simulink library "BMSI_lib"  (Simulink 7.5)
settings: Solver=ode45  StartTime=0.0  StopTime=10.0  RelTol=1e-3
values from neighbouring files (symbols this model uses):
  pBMSI_bool_HandShakeOverFlag_C = Simulink.Parameter    [BMSI_par.m]
  pBMSI_bool_InterLockOverFlag_C = Simulink.Parameter    [BMSI_par.m]
  pBMSI_bool_StnCfgStOverFlag_C = Simulink.Parameter    [BMSI_par.m]
  pBMSI_mV_DSPInterLowrRngThd_C = Simulink.Parameter    [BMSI_par.m]
  pBMSI_mV_DSPInterUpprRngThd_C = Simulink.Parameter    [BMSI_par.m]
  pBMSI_mV_InterlockDiffThd_C = Simulink.Parameter    [BMSI_par.m]
  pBMSI_mV_InterlockLowrRngThd_C = Simulink.Parameter    [BMSI_par.m]
  pBMSI_mV_InterlockUpprRngThd_C = Simulink.Parameter    [BMSI_par.m]
  pBMSI_pct_LoSOCThd_C = Simulink.Parameter    [BMSI_par.m]
  pBMSI_st_DCChrgrErrSt_C = Simulink.Parameter    [BMSI_par.m]
undefined symbols (not defined in the file or in its folder): ChrgHandShakeTyp, ChrgStationParCnfTyp, FAWBatInsMeasStsTyp, FAWBmsChrgStsTyp, FAWBmsContErrTyp, FAWBMSStsTyp, p_bool_dSPaceEnbl_C, p_bool_False_M, p_bool_True_M
libraries: BaseOperationLib_Browser x116, PES_CZ_FAW x15, simulink x1
(part 1 of 2)
settings Model: Creator=wuaibin  LastModifiedBy=wuaibin

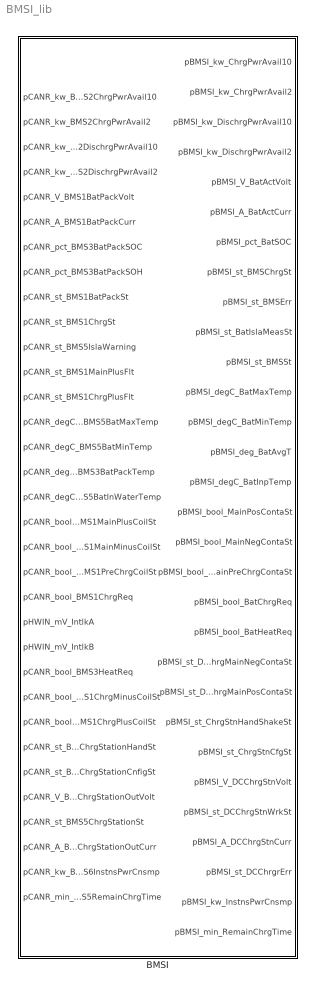
== system BMSI_lib ==
  BMSI : Subsystem  TreatAsAtomicUnit=on

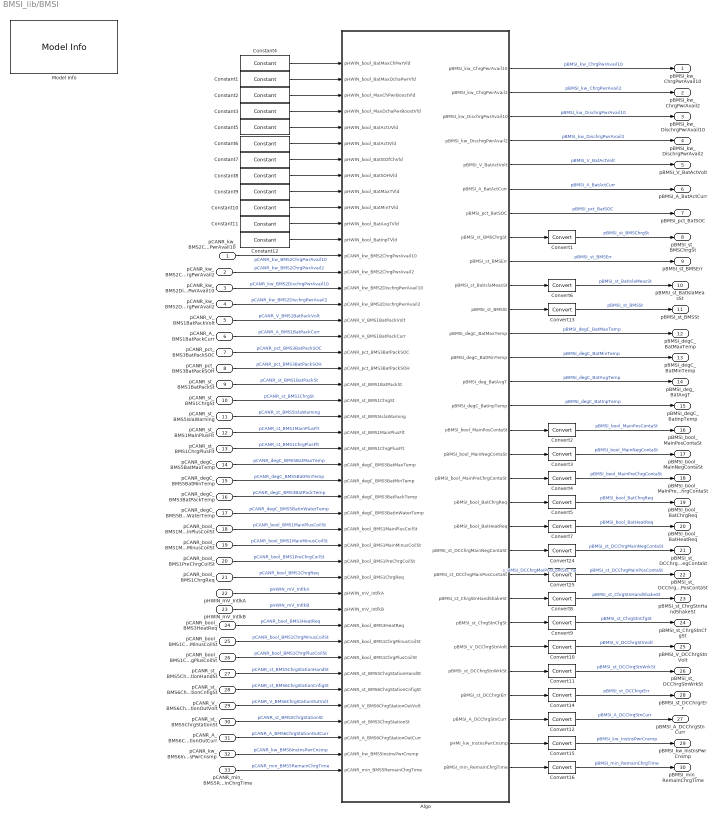
== system BMSI_lib/BMSI ==
  pCANR_kw_BMS2ChrgPwrAvail10 : Inport  OutDataType=fixdt(1, 16)  OutScaling=2^0
  pCANR_kw_BMS2ChrgPwrAvail2 : Inport  Port=2  OutDataType=fixdt(1, 16)  OutScaling=2^0
  pCANR_kw_BMS2DischrgPwrAvail10 : Inport  Port=3  OutDataType=fixdt(1, 16)  OutScaling=2^0
  pCANR_kw_BMS2DischrgPwrAvail2 : Inport  Port=4  OutDataType=fixdt(1, 16)  OutScaling=2^0
  pCANR_V_BMS1BatPackVolt : Inport  Port=5  OutDataType=fixdt(1, 16)  OutScaling=2^0
  pCANR_A_BMS1BatPackCurr : Inport  Port=6  OutDataType=fixdt(1, 16)  OutScaling=2^0
  pCANR_pct_BMS3BatPackSOC : Inport  Port=7  OutDataType=fixdt(1, 16)  OutScaling=2^0
  pCANR_pct_BMS3BatPackSOH : Inport  Port=8  OutDataType=fixdt(1, 16)  OutScaling=2^0
  pCANR_st_BMS1BatPackSt : Inport  Port=9  OutDataType=fixdt(1, 16)  OutScaling=2^0
  pCANR_st_BMS1ChrgSt : Inport  Port=10  OutDataType=fixdt(1, 16)  OutScaling=2^0
  pCANR_st_BMS5IslaWarning : Inport  Port=11  OutDataType=fixdt(1, 16)  OutScaling=2^0
  pCANR_st_BMS1MainPlusFlt : Inport  Port=12  OutDataType=fixdt(1, 16)  OutScaling=2^0
  pCANR_st_BMS1ChrgPlusFlt : Inport  Port=13  OutDataType=fixdt(1, 16)  OutScaling=2^0
  pCANR_degC_BMS5BatMaxTemp : Inport  Port=14  OutDataType=fixdt(1, 16)  OutScaling=2^0
  pCANR_degC_BMS5BatMinTemp : Inport  Port=15  OutDataType=fixdt(1, 16)  OutScaling=2^0
  pCANR_degC_BMS3BatPackTemp : Inport  Port=16  OutDataType=fixdt(1, 16)  OutScaling=2^0
  pCANR_degC_BMS5BatInWaterTemp : Inport  Port=17  OutDataType=fixdt(1, 16)  OutScaling=2^0
  pCANR_bool_BMS1MainPlusCoilSt : Inport  Port=18  OutDataType=fixdt(1, 16)  OutScaling=2^0
  pCANR_bool_BMS1MainMinusCoilSt : Inport  Port=19  OutDataType=fixdt(1, 16)  OutScaling=2^0
  pCANR_bool_BMS1PreChrgCoilSt : Inport  Port=20  OutDataType=fixdt(1, 16)  OutScaling=2^0
  pCANR_bool_BMS1ChrgReq : Inport  Port=21  OutDataType=fixdt(1, 16)  OutScaling=2^0
  pHWIN_mV_IntlkA : Inport  Port=22  OutDataType=fixdt(1, 16)  OutScaling=2^0
  pHWIN_mV_IntlkB : Inport  Port=23  OutDataType=fixdt(1, 16)  OutScaling=2^0
  pCANR_bool_BMS3HeatReq : Inport  Port=24  OutDataType=fixdt(1, 16)  OutScaling=2^0
  pCANR_bool_BMS1ChrgMinusCoilSt : Inport  Port=25  OutDataType=fixdt(1, 16)  OutScaling=2^0
  pCANR_bool_BMS1ChrgPlusCoilSt : Inport  Port=26  OutDataType=fixdt(1, 16)  OutScaling=2^0
  pCANR_st_BMS5ChrgStationHandSt : Inport  Port=27  OutDataType=fixdt(1, 16)  OutScaling=2^0
  pCANR_st_BMS6ChrgStationCnfigSt : Inport  Port=28  OutDataType=fixdt(1, 16)  OutScaling=2^0
  pCANR_V_BMS6ChrgStationOutVolt : Inport  Port=29  OutDataType=fixdt(1, 16)  OutScaling=2^0
  pCANR_st_BMS5ChrgStationSt : Inport  Port=30  OutDataType=fixdt(1, 16)  OutScaling=2^0
  pCANR_A_BMS6ChrgStationOutCurr : Inport  Port=31  OutDataType=fixdt(1, 16)  OutScaling=2^0
  pCANR_kw_BMS6InstnsPwrCnsmp : Inport  Port=32  OutDataType=fixdt(1, 16)  OutScaling=2^0
  pCANR_min_BMS5RemainChrgTime : Inport  Port=33  OutDataType=fixdt(1, 16)  OutScaling=2^0
  Algo : Subsystem
  Constant{1..12} (12 alike) : BaseOperationLib_Browser/Sources&Sinks/Constant  Value=p_bool_True_M  OutMin=[]  OutMax=[]  OutDataTypeMode=uint32  OutDataType=fixdt(1, 16)  ConRadixGroup=Use specified scaling  OutScaling=2^0  OutDataTypeStr=uint32
  Convert{1..16,24..25} (18 alike) : DataTypeConversion  OutDataType=fixdt(1, 16)  OutScaling=2^0
  Model Info : simulink/Model-Wide Utilities/Model Info  SystemSampleTime=-1  InitialBlockCM=None  BlockCM=None  Frame=on  DisplayStringWithTags=Model Info\nCreated: %<Created>\nCreator: %<Creator>  HorizontalTextAlignment=Center  LeftAlignmentValue=0.5  SourceBlockDiagram=HQEV_HCU  TagMaxNumber=20
  pBMSI_kw_ChrgPwrAvail10 : Outport  OutDataType=fixdt(1, 16)  OutScaling=2^0
  pBMSI_kw_ChrgPwrAvail2 : Outport  Port=2  OutDataType=fixdt(1, 16)  OutScaling=2^0
  pBMSI_kw_DischrgPwrAvail10 : Outport  Port=3  OutDataType=fixdt(1, 16)  OutScaling=2^0
  pBMSI_kw_DischrgPwrAvail2 : Outport  Port=4  OutDataType=fixdt(1, 16)  OutScaling=2^0
  pBMSI_V_BatActVolt : Outport  Port=5  OutDataType=fixdt(1, 16)  OutScaling=2^0
  pBMSI_A_BatActCurr : Outport  Port=6  OutDataType=fixdt(1, 16)  OutScaling=2^0
  pBMSI_pct_BatSOC : Outport  Port=7  OutDataType=fixdt(1, 16)  OutScaling=2^0
  pBMSI_st_BMSChrgSt : Outport  Port=8  OutDataType=fixdt(1, 16)  OutScaling=2^0
  pBMSI_st_BMSErr : Outport  Port=9  OutDataType=fixdt(1, 16)  OutScaling=2^0
  pBMSI_st_BatIslaMeasSt : Outport  Port=10  OutDataType=fixdt(1, 16)  OutScaling=2^0
  pBMSI_st_BMSSt : Outport  Port=11  OutDataType=fixdt(1, 16)  OutScaling=2^0
  pBMSI_degC_BatMaxTemp : Outport  Port=12  OutDataType=fixdt(1, 16)  OutScaling=2^0
  pBMSI_degC_BatMinTemp : Outport  Port=13  OutDataType=fixdt(1, 16)  OutScaling=2^0
  pBMSI_deg_BatAvgT : Outport  Port=14  OutDataType=fixdt(1, 16)  OutScaling=2^0
  pBMSI_degC_BatInpTemp : Outport  Port=15  OutDataType=fixdt(1, 16)  OutScaling=2^0
  pBMSI_bool_MainPosContaSt : Outport  Port=16  OutDataType=fixdt(1, 16)  OutScaling=2^0
  pBMSI_bool_MainNegContaSt : Outport  Port=17  OutDataType=fixdt(1, 16)  OutScaling=2^0
  pBMSI_bool_MainPreChrgContaSt : Outport  Port=18  OutDataType=fixdt(1, 16)  OutScaling=2^0
  pBMSI_bool_BatChrgReq : Outport  Port=19  OutDataType=fixdt(1, 16)  OutScaling=2^0
  pBMSI_bool_BatHeatReq : Outport  Port=20  OutDataType=fixdt(1, 16)  OutScaling=2^0
  pBMSI_st_DCChrgMainNegContaSt : Outport  Port=21  OutDataType=fixdt(1, 16)  OutScaling=2^0
  pBMSI_st_DCChrgMainPosContaSt : Outport  Port=22  OutDataType=fixdt(1, 16)  OutScaling=2^0
  pBMSI_st_ChrgStnHandShakeSt : Outport  Port=23  OutDataType=fixdt(1, 16)  OutScaling=2^0
  pBMSI_st_ChrgStnCfgSt : Outport  Port=24  OutDataType=fixdt(1, 16)  OutScaling=2^0
  pBMSI_V_DCChrgStnVolt : Outport  Port=25  OutDataType=fixdt(1, 16)  OutScaling=2^0
  pBMSI_st_DCChrgStnWrkSt : Outport  Port=26  OutDataType=fixdt(1, 16)  OutScaling=2^0
  pBMSI_A_DCChrgStnCurr : Outport  Port=27  OutDataType=fixdt(1, 16)  OutScaling=2^0
  pBMSI_st_DCChrgrErr : Outport  Port=28  OutDataType=fixdt(1, 16)  OutScaling=2^0
  pBMSI_kw_InstnsPwrCnsmp : Outport  Port=29  OutDataType=fixdt(1, 16)  OutScaling=2^0
  pBMSI_min_RemainChrgTime : Outport  Port=30  OutDataType=fixdt(1, 16)  OutScaling=2^0
  wires:
  Algo/11(pBMSI_st_BMSSt) -> Convert13/1
  Algo/10(pBMSI_st_BatIslaMeasSt) -> Convert6/1
  Algo/28(pBMSI_A_DCChrgStnCurr) -> Convert12/1
  pCANR_st_BMS1ChrgPlusFlt/1 -> Algo/25(pCANR_st_BMS1ChrgPlusFlt)  "pCANR_st_BMS1ChrgPlusFlt"
  pCANR_st_BMS1MainPlusFlt/1 -> Algo/24(pCANR_st_BMS1MainPlusFlt)  "pCANR_st_BMS1MainPlusFlt"
  Algo/30(pBMSI_min_RemainChrgTime) -> Convert16/1
  pCANR_min_BMS5RemainChrgTime/1 -> Algo/45(pCANR_min_BMS5RemainChrgTime)  "pCANR_min_BMS5RemainChrgTime"
  Convert16/1 -> pBMSI_min_RemainChrgTime/1  "pBMSI_min_RemainChrgTime"
  Convert15/1 -> pBMSI_kw_InstnsPwrCnsmp/1  "pBMSI_kw_InstnsPwrCnsmp"
  Algo/29(pHMI_kw_InstnsPwrCnsmp) -> Convert15/1
  pCANR_kw_BMS6InstnsPwrCnsmp/1 -> Algo/44(pCANR_kw_BMS5InstnsPwrCnsmp)  "pCANR_kw_BMS6InstnsPwrCnsmp"
  Convert25/1 -> pBMSI_st_DCChrgMainPosContaSt/1  "pBMSI_st_DCChrgMainPosContaSt"
  Convert12/1 -> pBMSI_A_DCChrgStnCurr/1  "pBMSI_A_DCChrgStnCurr"
  Convert11/1 -> pBMSI_st_DCChrgStnWrkSt/1  "pBMSI_st_DCChrgStnWrkSt"
  Convert10/1 -> pBMSI_V_DCChrgStnVolt/1  "pBMSI_V_DCChrgStnVolt"
  Convert9/1 -> pBMSI_st_ChrgStnCfgSt/1  "pBMSI_st_ChrgStnCfgSt"
  Convert8/1 -> pBMSI_st_ChrgStnHandShakeSt/1  "pBMSI_st_ChrgStnHandShakeSt"
  Convert7/1 -> pBMSI_bool_BatHeatReq/1  "pBMSI_bool_BatHeatReq"
  Convert6/1 -> pBMSI_st_BatIslaMeasSt/1  "pBMSI_st_BatIslaMeasSt"
  Convert5/1 -> pBMSI_bool_BatChrgReq/1  "pBMSI_bool_BatChrgReq"
  Convert4/1 -> pBMSI_bool_MainPreChrgContaSt/1  "pBMSI_bool_MainPreChrgContaSt"
  Convert3/1 -> pBMSI_bool_MainNegContaSt/1  "pBMSI_bool_MainNegContaSt"
  Convert2/1 -> pBMSI_bool_MainPosContaSt/1  "pBMSI_bool_MainPosContaSt"
  Convert1/1 -> pBMSI_st_BMSChrgSt/1  "pBMSI_st_BMSChrgSt"
  pCANR_A_BMS6ChrgStationOutCurr/1 -> Algo/43(pCANR_A_BMS6ChrgStationOutCurr)  "pCANR_A_BMS6ChrgStationOutCurr"
  pCANR_st_BMS5ChrgStationSt/1 -> Algo/42(pCANR_st_BMS5ChrgStationSt)  "pCANR_st_BMS5ChrgStationSt"
  pCANR_V_BMS6ChrgStationOutVolt/1 -> Algo/41(pCANR_V_BMS6ChrgStationOutVolt)  "pCANR_V_BMS6ChrgStationOutVolt"
  pCANR_st_BMS6ChrgStationCnfigSt/1 -> Algo/40(pCANR_st_BMS6ChrgStationCnfigSt)  "pCANR_st_BMS6ChrgStationCnfigSt"
  pCANR_st_BMS5ChrgStationHandSt/1 -> Algo/39(pCANR_st_BMS5ChrgStationHandSt)  "pCANR_st_BMS5ChrgStationHandSt"
  pCANR_bool_BMS1ChrgPlusCoilSt/1 -> Algo/38(pCANR_bool_BMS1ChrgPlusCoilSt)  "pCANR_bool_BMS1ChrgPlusCoilSt"
  pCANR_bool_BMS1ChrgMinusCoilSt/1 -> Algo/37(pCANR_bool_BMS1ChrgMinusCoilSt)  "pCANR_bool_BMS1ChrgMinusCoilSt"
  pCANR_bool_BMS3HeatReq/1 -> Algo/36(pCANR_bool_BMS3HeatReq)  "pCANR_bool_BMS3HeatReq"
  pCANR_kw_BMS2ChrgPwrAvail10/1 -> Algo/13(pCANR_kw_BMS2ChrgPwrAvail10)  "pCANR_kw_BMS2ChrgPwrAvail10"
  Constant4/1 -> Algo/1(pHWIN_bool_BatMaxChPwrVld)
  Constant1/1 -> Algo/2(pHWIN_bool_BatMaxDchaPwrVld)
  Constant2/1 -> Algo/3(pHWIN_bool_MaxChPwrBoostVld)
  Constant3/1 -> Algo/4(pHWIN_bool_MaxDchaPwrBoostVld)
  Constant5/1 -> Algo/5(pHWIN_bool_BatActUVld)
  Constant6/1 -> Algo/6(pHWIN_bool_BatActIVld)
  Constant7/1 -> Algo/7(pHWIN_bool_BatStOfChVld)
  Constant8/1 -> Algo/8(pHWIN_bool_BatSOHVld)
  Constant9/1 -> Algo/9(pHWIN_bool_BatMaxTVld)
  Constant10/1 -> Algo/10(pHWIN_bool_BatMinTVld)
  Constant11/1 -> Algo/11(pHWIN_bool_BatAvgTVld)
  Constant12/1 -> Algo/12(pHWIN_bool_BatInpTVld)
  pCANR_kw_BMS2ChrgPwrAvail2/1 -> Algo/14(pCANR_kw_BMS2ChrgPwrAvail2)  "pCANR_kw_BMS2ChrgPwrAvail2"
  pCANR_kw_BMS2DischrgPwrAvail10/1 -> Algo/15(pCANR_kw_BMS2DischrgPwrAvail10)  "pCANR_kw_BMS2DischrgPwrAvail10"
  pCANR_kw_BMS2DischrgPwrAvail2/1 -> Algo/16(pCANR_kw_BMS2DischrgPwrAvail2)  "pCANR_kw_BMS2DischrgPwrAvail2"
  pCANR_V_BMS1BatPackVolt/1 -> Algo/17(pCANR_V_BMS1BatPackVolt)  "pCANR_V_BMS1BatPackVolt"
  pCANR_A_BMS1BatPackCurr/1 -> Algo/18(pCANR_A_BMS1BatPackCurr)  "pCANR_A_BMS1BatPackCurr"
  pCANR_pct_BMS3BatPackSOC/1 -> Algo/19(pCANR_pct_BMS3BatPackSOC)  "pCANR_pct_BMS3BatPackSOC"
  pCANR_pct_BMS3BatPackSOH/1 -> Algo/20(pCANR_pct_BMS3BatPackSOH)  "pCANR_pct_BMS3BatPackSOH"
  pCANR_st_BMS1BatPackSt/1 -> Algo/21(pCANR_st_BMS1BatPackSt)  "pCANR_st_BMS1BatPackSt"
  pCANR_st_BMS1ChrgSt/1 -> Algo/22(pCANR_st_BMS1ChrgSt)  "pCANR_st_BMS1ChrgSt"
  pCANR_st_BMS5IslaWarning/1 -> Algo/23(pCANR_st_BMS5IslaWarning)  "pCANR_st_BMS5IslaWarning"
  pCANR_degC_BMS5BatMaxTemp/1 -> Algo/26(pCANR_degC_BMS5BatMaxTemp)  "pCANR_degC_BMS5BatMaxTemp"
  pCANR_degC_BMS5BatMinTemp/1 -> Algo/27(pCANR_degC_BMS5BatMinTemp)  "pCANR_degC_BMS5BatMinTemp"
  pCANR_degC_BMS3BatPackTemp/1 -> Algo/28(pCANR_degC_BMS3BatPackTemp)  "pCANR_degC_BMS3BatPackTemp"
  pCANR_degC_BMS5BatInWaterTemp/1 -> Algo/29(pCANR_degC_BMS5BatInWaterTemp)  "pCANR_degC_BMS5BatInWaterTemp"
  pCANR_bool_BMS1MainPlusCoilSt/1 -> Algo/30(pCANR_bool_BMS1MainPlusCoilSt)  "pCANR_bool_BMS1MainPlusCoilSt"
  pCANR_bool_BMS1MainMinusCoilSt/1 -> Algo/31(pCANR_bool_BMS1MainMinusCoilSt)  "pCANR_bool_BMS1MainMinusCoilSt"
  pCANR_bool_BMS1PreChrgCoilSt/1 -> Algo/32(pCANR_bool_BMS1PreChrgCoilSt)  "pCANR_bool_BMS1PreChrgCoilSt"
  pCANR_bool_BMS1ChrgReq/1 -> Algo/33(pCANR_bool_BMS1ChrgReq)  "pCANR_bool_BMS1ChrgReq"
  pHWIN_mV_IntlkA/1 -> Algo/34(pHWIN_mV_IntlkA)  "pHWIN_mV_IntlkA"
  pHWIN_mV_IntlkB/1 -> Algo/35(pHWIN_mV_IntlkB)  "pHWIN_mV_IntlkB"
  Algo/26(pBMSI_st_DCChrgStnWrkSt) -> Convert11/1
  Algo/25(pBMSI_V_DCChrgStnVolt) -> Convert10/1
  Convert24/1 -> pBMSI_st_DCChrgMainNegContaSt/1  "pBMSI_st_DCChrgMainNegContaSt"
  Algo/24(pBMSI_st_ChrgStnCfgSt) -> Convert9/1
  Algo/23(pBMSI_st_ChrgStnHandShakeSt) -> Convert8/1
  Algo/22(pBMSI_st_DCChrgMainPosContaSt) -> Convert25/1  "s_BMSI_DCChrgMaiPosContSts_na"
  Algo/21(pBMSI_st_DCChrgMainNegContaSt) -> Convert24/1
  Algo/20(pBMSI_bool_BatHeatReq) -> Convert7/1
  Algo/1(pBMSI_kw_ChrgPwrAvail10) -> pBMSI_kw_ChrgPwrAvail10/1  "pBMSI_kw_ChrgPwrAvail10"
  Algo/3(pBMSI_kw_DischrgPwrAvail10) -> pBMSI_kw_DischrgPwrAvail10/1  "pBMSI_kw_DischrgPwrAvail10"
  Algo/5(pBMSI_V_BatActVolt) -> pBMSI_V_BatActVolt/1  "pBMSI_V_BatActVolt"
  Algo/6(pBMSI_A_BatActCurr) -> pBMSI_A_BatActCurr/1  "pBMSI_A_BatActCurr"
  Algo/7(pBMSI_pct_BatSOC) -> pBMSI_pct_BatSOC/1  "pBMSI_pct_BatSOC"
  Algo/8(pBMSI_st_BMSChrgSt) -> Convert1/1
  Algo/12(pBMSI_degC_BatMaxTemp) -> pBMSI_degC_BatMaxTemp/1  "pBMSI_degC_BatMaxTemp"
  Algo/13(pBMSI_degC_BatMinTemp) -> pBMSI_degC_BatMinTemp/1  "pBMSI_degC_BatMinTemp"
  Algo/14(pBMSI_deg_BatAvgT) -> pBMSI_deg_BatAvgT/1  "pBMSI_degC_BatAvgTemp"
  Algo/15(pBMSI_degC_BatInpTemp) -> pBMSI_degC_BatInpTemp/1  "pBMSI_degC_BatInpTemp"
  Algo/9(pBMSI_st_BMSErr) -> pBMSI_st_BMSErr/1  "pBMSI_st_BMSErr"
  Algo/16(pBMSI_bool_MainPosContaSt) -> Convert2/1
  Algo/17(pBMSI_bool_MainNegContaSt) -> Convert3/1
  Algo/18(pBMSI_bool_MainPreChrgContaSt) -> Convert4/1
  Algo/19(pBMSI_bool_BatChrgReq) -> Convert5/1
  Algo/2(pBMSI_kw_ChrgPwrAvail2) -> pBMSI_kw_ChrgPwrAvail2/1  "pBMSI_kw_ChrgPwrAvail2"
  Algo/4(pBMSI_kw_DischrgPwrAvail2) -> pBMSI_kw_DischrgPwrAvail2/1  "pBMSI_kw_DischrgPwrAvail2"
  Convert13/1 -> pBMSI_st_BMSSt/1  "pBMSI_st_BMSSt"
  Algo/27(pBMSI_st_DCChrgrErr) -> Convert14/1
  Convert14/1 -> pBMSI_st_DCChrgrErr/1  "pBMSI_st_DCChrgrErr"

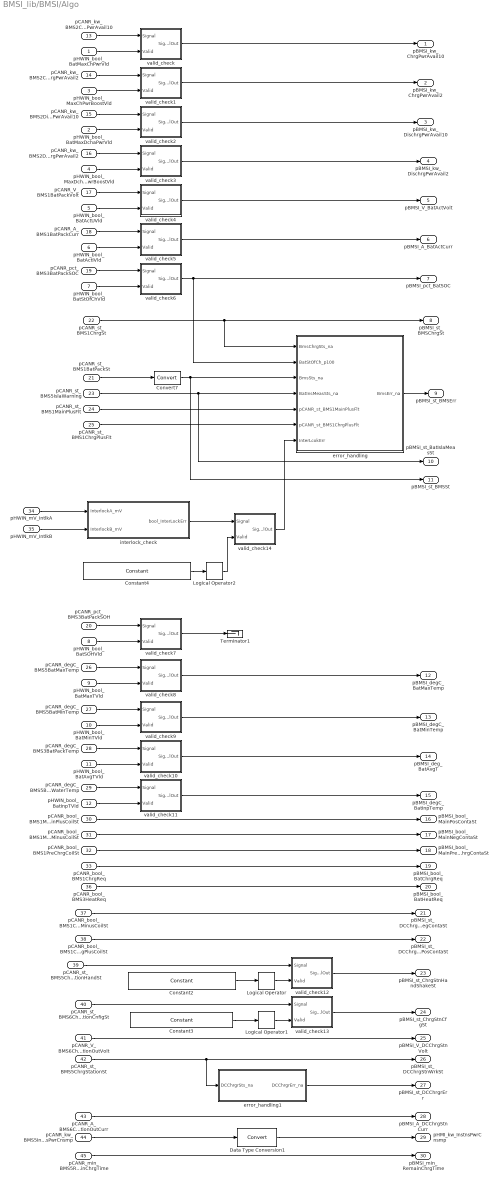
== system BMSI_lib/BMSI/Algo ==
  pHWIN_bool_BatMaxChPwrVld : Inport  OutDataType=fixdt(1, 16)  OutScaling=2^0
  pHWIN_bool_BatMaxDchaPwrVld : Inport  Port=2  OutDataType=fixdt(1, 16)  OutScaling=2^0
  pHWIN_bool_MaxChPwrBoostVld : Inport  Port=3  OutDataType=fixdt(1, 16)  OutScaling=2^0
  pHWIN_bool_MaxDchaPwrBoostVld : Inport  Port=4  OutDataType=fixdt(1, 16)  OutScaling=2^0
  pHWIN_bool_BatActUVld : Inport  Port=5  OutDataType=fixdt(1, 16)  OutScaling=2^0
  pHWIN_bool_BatActIVld : Inport  Port=6  OutDataType=fixdt(1, 16)  OutScaling=2^0
  pHWIN_bool_BatStOfChVld : Inport  Port=7  OutDataType=fixdt(1, 16)  OutScaling=2^0
  pHWIN_bool_BatSOHVld : Inport  Port=8  OutDataType=fixdt(1, 16)  OutScaling=2^0
  pHWIN_bool_BatMaxTVld : Inport  Port=9  OutDataType=fixdt(1, 16)  OutScaling=2^0
  pHWIN_bool_BatMinTVld : Inport  Port=10  OutDataType=fixdt(1, 16)  OutScaling=2^0
  pHWIN_bool_BatAvgTVld : Inport  Port=11  OutDataType=fixdt(1, 16)  OutScaling=2^0
  pHWIN_bool_BatInpTVld : Inport  Port=12  OutDataType=fixdt(1, 16)  OutScaling=2^0
  pCANR_kw_BMS2ChrgPwrAvail10 : Inport  Port=13  OutDataType=fixdt(1, 16)  OutScaling=2^0
  pCANR_kw_BMS2ChrgPwrAvail2 : Inport  Port=14  OutDataType=fixdt(1, 16)  OutScaling=2^0
  pCANR_kw_BMS2DischrgPwrAvail10 : Inport  Port=15  OutDataType=fixdt(1, 16)  OutScaling=2^0
  pCANR_kw_BMS2DischrgPwrAvail2 : Inport  Port=16  OutDataType=fixdt(1, 16)  OutScaling=2^0
  pCANR_V_BMS1BatPackVolt : Inport  Port=17  OutDataType=fixdt(1, 16)  OutScaling=2^0
  pCANR_A_BMS1BatPackCurr : Inport  Port=18  OutDataType=fixdt(1, 16)  OutScaling=2^0
  pCANR_pct_BMS3BatPackSOC : Inport  Port=19  OutDataType=fixdt(1, 16)  OutScaling=2^0
  pCANR_pct_BMS3BatPackSOH : Inport  Port=20  OutDataType=fixdt(1, 16)  OutScaling=2^0
  pCANR_st_BMS1BatPackSt : Inport  Port=21  OutDataType=fixdt(1, 16)  OutScaling=2^0
  pCANR_st_BMS1ChrgSt : Inport  Port=22  OutDataType=fixdt(1, 16)  OutScaling=2^0
  pCANR_st_BMS5IslaWarning : Inport  Port=23  OutDataType=fixdt(1, 16)  OutScaling=2^0
  pCANR_st_BMS1MainPlusFlt : Inport  Port=24  OutDataType=fixdt(1, 16)  OutScaling=2^0
  pCANR_st_BMS1ChrgPlusFlt : Inport  Port=25  OutDataType=fixdt(1, 16)  OutScaling=2^0
  pCANR_degC_BMS5BatMaxTemp : Inport  Port=26  OutDataType=fixdt(1, 16)  OutScaling=2^0
  pCANR_degC_BMS5BatMinTemp : Inport  Port=27  OutDataType=fixdt(1, 16)  OutScaling=2^0
  pCANR_degC_BMS3BatPackTemp : Inport  Port=28  OutDataType=fixdt(1, 16)  OutScaling=2^0
  pCANR_degC_BMS5BatInWaterTemp : Inport  Port=29  OutDataType=fixdt(1, 16)  OutScaling=2^0
  pCANR_bool_BMS1MainPlusCoilSt : Inport  Port=30  OutDataType=fixdt(1, 16)  OutScaling=2^0
  pCANR_bool_BMS1MainMinusCoilSt : Inport  Port=31  OutDataType=fixdt(1, 16)  OutScaling=2^0
  pCANR_bool_BMS1PreChrgCoilSt : Inport  Port=32  OutDataType=fixdt(1, 16)  OutScaling=2^0
  pCANR_bool_BMS1ChrgReq : Inport  Port=33  OutDataType=fixdt(1, 16)  OutScaling=2^0
  pHWIN_mV_IntlkA : Inport  Port=34  OutDataType=fixdt(1, 16)  OutScaling=2^0
  pHWIN_mV_IntlkB : Inport  Port=35  OutDataType=fixdt(1, 16)  OutScaling=2^0
  pCANR_bool_BMS3HeatReq : Inport  Port=36  OutDataType=fixdt(1, 16)  OutScaling=2^0
  pCANR_bool_BMS1ChrgMinusCoilSt : Inport  Port=37  OutDataType=fixdt(1, 16)  OutScaling=2^0
  pCANR_bool_BMS1ChrgPlusCoilSt : Inport  Port=38  OutDataType=fixdt(1, 16)  OutScaling=2^0
  pCANR_st_BMS5ChrgStationHandSt : Inport  Port=39  OutDataType=fixdt(1, 16)  OutScaling=2^0
  pCANR_st_BMS6ChrgStationCnfigSt : Inport  Port=40  OutDataType=fixdt(1, 16)  OutScaling=2^0
  pCANR_V_BMS6ChrgStationOutVolt : Inport  Port=41  OutDataType=fixdt(1, 16)  OutScaling=2^0
  pCANR_st_BMS5ChrgStationSt : Inport  Port=42  OutDataType=fixdt(1, 16)  OutScaling=2^0
  pCANR_A_BMS6ChrgStationOutCurr : Inport  Port=43  OutDataType=fixdt(1, 16)  OutScaling=2^0
  pCANR_kw_BMS5InstnsPwrCnsmp : Inport  Port=44  OutDataType=fixdt(1, 16)  OutScaling=2^0
  pCANR_min_BMS5RemainChrgTime : Inport  Port=45  OutDataType=fixdt(1, 16)  OutScaling=2^0
  Constant2 : BaseOperationLib_Browser/Sources&Sinks/Constant  Value=pBMSI_bool_HandShakeOverFlag_C  OutMin=[]  OutMax=[]  OutDataType=fixdt(1, 16)  ConRadixGroup=Use specified scaling  OutScaling=2^0  OutDataTypeStr=Inherit: Inherit from 'Constant value'
  Constant3 : BaseOperationLib_Browser/Sources&Sinks/Constant  Value=pBMSI_bool_StnCfgStOverFlag_C  OutMin=[]  OutMax=[]  OutDataType=fixdt(1, 16)  ConRadixGroup=Use specified scaling  OutScaling=2^0  OutDataTypeStr=Inherit: Inherit from 'Constant value'
  Constant4 : BaseOperationLib_Browser/Sources&Sinks/Constant  Value=pBMSI_bool_InterLockOverFlag_C  OutMin=[]  OutMax=[]  OutDataType=fixdt(1, 16)  ConRadixGroup=Use specified scaling  OutScaling=2^0  OutDataTypeStr=Inherit: Inherit from 'Constant value'
  Convert7 : DataTypeConversion  OutDataType=fixdt(1, 16)  OutScaling=2^0
  Data Type Conversion1 : DataTypeConversion  OutDataType=fixdt(1, 16)  OutScaling=2^0
  Logical Operator : BaseOperationLib_Browser/Logic Operations Changed/Logical Operator  Operator=NOT  Inputs=2  AllPortsSameDT=on  OutDataTypeMode=Specify via dialog  LogicDataType=PDT_Bool  OutDataTypeStr=PDT_Bool
  Logical Operator1 : BaseOperationLib_Browser/Logic Operations Changed/Logical Operator  Operator=NOT  Inputs=2  AllPortsSameDT=on  OutDataTypeMode=Specify via dialog  LogicDataType=PDT_Bool  OutDataTypeStr=PDT_Bool
  Logical Operator2 : BaseOperationLib_Browser/Logic Operations Changed/Logical Operator  Operator=NOT  Inputs=2  AllPortsSameDT=on  OutDataTypeMode=Specify via dialog  LogicDataType=PDT_Bool  OutDataTypeStr=PDT_Bool
  Terminator1 : Terminator
  error_handling : Subsystem
  error_handling1 : Subsystem
  interlock_check : Subsystem
  valid_check : Subsystem  mask(Validity check      ){init=0}
      mask prompts: init "Init value"
      mask help:
      | Block checks, if the signal is valid. If not, signal is replaced by its
      | last valid value.
      mask Help:
      | Block checks, if the signal is valid. If not, signal is replaced by its
      | last valid value.
  valid_check1 : Subsystem  mask(Validity check      ){init=0}
      mask prompts: init "Init value"
      mask help:
      | Block checks, if the signal is valid. If not, signal is replaced by its
      | last valid value.
      mask Help:
      | Block checks, if the signal is valid. If not, signal is replaced by its
      | last valid value.
  valid_check10 : Subsystem  mask(Validity check      ){init=20}
      mask prompts: init "Init value"
      mask help:
      | Block checks, if the signal is valid. If not, signal is replaced by its
      | last valid value.
      mask Help:
      | Block checks, if the signal is valid. If not, signal is replaced by its
      | last valid value.
  valid_check11 : Subsystem  mask(Validity check      ){init=20}
      mask prompts: init "Init value"
      mask help:
      | Block checks, if the signal is valid. If not, signal is replaced by its
      | last valid value.
      mask Help:
      | Block checks, if the signal is valid. If not, signal is replaced by its
      | last valid value.
  valid_check12 : Subsystem  mask(Validity check      ){init=uint8(ChrgHandShakeTyp.shake_Success)}
      mask prompts: init "Init value"
      mask help:
      | Block checks, if the signal is valid. If not, signal is replaced by its
      | last valid value.
      mask Help:
      | Block checks, if the signal is valid. If not, signal is replaced by its
      | last valid value.
  valid_check13 : Subsystem  mask(Validity check      ){init=uint8(ChrgStationParCnfTyp.ParConfig_Success)}
      mask prompts: init "Init value"
      mask help:
      | Block checks, if the signal is valid. If not, signal is replaced by its
      | last valid value.
      mask Help:
      | Block checks, if the signal is valid. If not, signal is replaced by its
      | last valid value.
  valid_check14 : Subsystem  mask(Validity check      ){init=p_bool_False_M}
      mask prompts: init "Init value"
      mask help:
      | Block checks, if the signal is valid. If not, signal is replaced by its
      | last valid value.
      mask Help:
      | Block checks, if the signal is valid. If not, signal is replaced by its
      | last valid value.
  valid_check2 : Subsystem  mask(Validity check      ){init=0}
      mask prompts: init "Init value"
      mask help:
      | Block checks, if the signal is valid. If not, signal is replaced by its
      | last valid value.
      mask Help:
      | Block checks, if the signal is valid. If not, signal is replaced by its
      | last valid value.
  valid_check3 : Subsystem  mask(Validity check      ){init=0}
      mask prompts: init "Init value"
      mask help:
      | Block checks, if the signal is valid. If not, signal is replaced by its
      | last valid value.
      mask Help:
      | Block checks, if the signal is valid. If not, signal is replaced by its
      | last valid value.
  valid_check4 : Subsystem  mask(Validity check      ){init=0}
      mask prompts: init "Init value"
      mask help:
      | Block checks, if the signal is valid. If not, signal is replaced by its
      | last valid value.
      mask Help:
      | Block checks, if the signal is valid. If not, signal is replaced by its
      | last valid value.
  valid_check5 : Subsystem  mask(Validity check      ){init=0}
      mask prompts: init "Init value"
      mask help:
      | Block checks, if the signal is valid. If not, signal is replaced by its
      | last valid value.
      mask Help:
      | Block checks, if the signal is valid. If not, signal is replaced by its
      | last valid value.
  valid_check6 : Subsystem  mask(Validity check      ){init=0}
      mask prompts: init "Init value"
      mask help:
      | Block checks, if the signal is valid. If not, signal is replaced by its
      | last valid value.
      mask Help:
      | Block checks, if the signal is valid. If not, signal is replaced by its
      | last valid value.
  valid_check7 : Subsystem  mask(Validity check      ){init=0}
      mask prompts: init "Init value"
      mask help:
      | Block checks, if the signal is valid. If not, signal is replaced by its
      | last valid value.
      mask Help:
      | Block checks, if the signal is valid. If not, signal is replaced by its
      | last valid value.
  valid_check8 : Subsystem  mask(Validity check      ){init=20}
      mask prompts: init "Init value"
      mask help:
      | Block checks, if the signal is valid. If not, signal is replaced by its
      | last valid value.
      mask Help:
      | Block checks, if the signal is valid. If not, signal is replaced by its
      | last valid value.
  valid_check9 : Subsystem  mask(Validity check      ){init=20}
      mask prompts: init "Init value"
      mask help:
      | Block checks, if the signal is valid. If not, signal is replaced by its
      | last valid value.
      mask Help:
      | Block checks, if the signal is valid. If not, signal is replaced by its
      | last valid value.
  pBMSI_kw_ChrgPwrAvail10 : Outport  OutDataType=fixdt(1, 16)  OutScaling=2^0
  pBMSI_kw_ChrgPwrAvail2 : Outport  Port=2  OutDataType=fixdt(1, 16)  OutScaling=2^0
  pBMSI_kw_DischrgPwrAvail10 : Outport  Port=3  OutDataType=fixdt(1, 16)  OutScaling=2^0
  pBMSI_kw_DischrgPwrAvail2 : Outport  Port=4  OutDataType=fixdt(1, 16)  OutScaling=2^0
  pBMSI_V_BatActVolt : Outport  Port=5  OutDataType=fixdt(1, 16)  OutScaling=2^0
  pBMSI_A_BatActCurr : Outport  Port=6  OutDataType=fixdt(1, 16)  OutScaling=2^0
  pBMSI_pct_BatSOC : Outport  Port=7  OutDataType=fixdt(1, 16)  OutScaling=2^0
  pBMSI_st_BMSChrgSt : Outport  Port=8  OutDataType=fixdt(1, 16)  OutScaling=2^0
  pBMSI_st_BMSErr : Outport  Port=9  OutDataType=fixdt(1, 16)  OutScaling=2^0
  pBMSI_st_BatIslaMeasSt : Outport  Port=10  OutDataType=fixdt(1, 16)  OutScaling=2^0
  pBMSI_st_BMSSt : Outport  Port=11  OutDataType=fixdt(1, 16)  OutScaling=2^0
  pBMSI_degC_BatMaxTemp : Outport  Port=12  OutDataType=fixdt(1, 16)  OutScaling=2^0
  pBMSI_degC_BatMinTemp : Outport  Port=13  OutDataType=fixdt(1, 16)  OutScaling=2^0
  pBMSI_deg_BatAvgT : Outport  Port=14  OutDataType=fixdt(1, 16)  OutScaling=2^0
  pBMSI_degC_BatInpTemp : Outport  Port=15  OutDataType=fixdt(1, 16)  OutScaling=2^0
  pBMSI_bool_MainPosContaSt : Outport  Port=16  OutDataType=fixdt(1, 16)  OutScaling=2^0
  pBMSI_bool_MainNegContaSt : Outport  Port=17  OutDataType=fixdt(1, 16)  OutScaling=2^0
  pBMSI_bool_MainPreChrgContaSt : Outport  Port=18  OutDataType=fixdt(1, 16)  OutScaling=2^0
  pBMSI_bool_BatChrgReq : Outport  Port=19  OutDataType=fixdt(1, 16)  OutScaling=2^0
  pBMSI_bool_BatHeatReq : Outport  Port=20  OutDataType=fixdt(1, 16)  OutScaling=2^0
  pBMSI_st_DCChrgMainNegContaSt : Outport  Port=21  OutDataType=fixdt(1, 16)  OutScaling=2^0
  pBMSI_st_DCChrgMainPosContaSt : Outport  Port=22  OutDataType=fixdt(1, 16)  OutScaling=2^0
  pBMSI_st_ChrgStnHandShakeSt : Outport  Port=23  OutDataType=fixdt(1, 16)  OutScaling=2^0
  pBMSI_st_ChrgStnCfgSt : Outport  Port=24  OutDataType=fixdt(1, 16)  OutScaling=2^0
  pBMSI_V_DCChrgStnVolt : Outport  Port=25  OutDataType=fixdt(1, 16)  OutScaling=2^0
  pBMSI_st_DCChrgStnWrkSt : Outport  Port=26  OutDataType=fixdt(1, 16)  OutScaling=2^0
  pBMSI_st_DCChrgrErr : Outport  Port=27  OutDataType=fixdt(1, 16)  OutScaling=2^0
  pBMSI_A_DCChrgStnCurr : Outport  Port=28  OutDataType=fixdt(1, 16)  OutScaling=2^0
  pHMI_kw_InstnsPwrCnsmp : Outport  Port=29  OutDataType=fixdt(1, 16)  OutScaling=2^0
  pBMSI_min_RemainChrgTime : Outport  Port=30  OutDataType=fixdt(1, 16)  OutScaling=2^0
  wires:
  Logical Operator2/1 -> valid_check14/2(Valid)
  Constant4/1 -> Logical Operator2/1
  Constant3/1 -> Logical Operator1/1
  Logical Operator1/1 -> valid_check13/2(Valid)
  Logical Operator/1 -> valid_check12/2(Valid)
  Constant2/1 -> Logical Operator/1
  interlock_check/1(bool_InterLockErr) -> valid_check14/1(Signal)
  valid_check14/1(SignalOut) -> error_handling/7(InterLcokErr)
  pCANR_st_BMS5ChrgStationHandSt/1 -> valid_check12/1(Signal)
  valid_check12/1(SignalOut) -> pBMSI_st_ChrgStnHandShakeSt/1
  pCANR_st_BMS6ChrgStationCnfigSt/1 -> valid_check13/1(Signal)
  valid_check13/1(SignalOut) -> pBMSI_st_ChrgStnCfgSt/1
  pCANR_st_BMS1MainPlusFlt/1 -> error_handling/5(pCANR_st_BMS1MainPlusFlt)
  pCANR_st_BMS1ChrgPlusFlt/1 -> error_handling/6(pCANR_st_BMS1ChrgPlusFlt)
  pCANR_min_BMS5RemainChrgTime/1 -> pBMSI_min_RemainChrgTime/1
  Data Type Conversion1/1 -> pHMI_kw_InstnsPwrCnsmp/1
  pCANR_kw_BMS5InstnsPwrCnsmp/1 -> Data Type Conversion1/1
  pCANR_A_BMS6ChrgStationOutCurr/1 -> pBMSI_A_DCChrgStnCurr/1
  pCANR_st_BMS5ChrgStationSt/1 -> pBMSI_st_DCChrgStnWrkSt/1, error_handling1/1(DCChrgrSts_na)
  pCANR_V_BMS6ChrgStationOutVolt/1 -> pBMSI_V_DCChrgStnVolt/1
  pCANR_bool_BMS1ChrgPlusCoilSt/1 -> pBMSI_st_DCChrgMainPosContaSt/1
  pCANR_bool_BMS1ChrgMinusCoilSt/1 -> pBMSI_st_DCChrgMainNegContaSt/1
  pCANR_bool_BMS3HeatReq/1 -> pBMSI_bool_BatHeatReq/1
  pHWIN_bool_BatActIVld/1 -> valid_check5/2(Valid)
  pHWIN_bool_BatStOfChVld/1 -> valid_check6/2(Valid)
  valid_check/1(SignalOut) -> pBMSI_kw_ChrgPwrAvail10/1
  valid_check1/1(SignalOut) -> pBMSI_kw_ChrgPwrAvail2/1
  valid_check2/1(SignalOut) -> pBMSI_kw_DischrgPwrAvail10/1
  valid_check3/1(SignalOut) -> pBMSI_kw_DischrgPwrAvail2/1
  valid_check4/1(SignalOut) -> pBMSI_V_BatActVolt/1
  pCANR_kw_BMS2ChrgPwrAvail10/1 -> valid_check/1(Signal)
  pHWIN_bool_BatMaxChPwrVld/1 -> valid_check/2(Valid)
  pHWIN_bool_MaxDchaPwrBoostVld/1 -> valid_check3/2(Valid)
  pHWIN_bool_MaxChPwrBoostVld/1 -> valid_check1/2(Valid)
  pHWIN_bool_BatMaxDchaPwrVld/1 -> valid_check2/2(Valid)
  pHWIN_bool_BatActUVld/1 -> valid_check4/2(Valid)
  pCANR_V_BMS1BatPackVolt/1 -> valid_check4/1(Signal)
  pCANR_kw_BMS2DischrgPwrAvail10/1 -> valid_check2/1(Signal)
  pCANR_kw_BMS2DischrgPwrAvail2/1 -> valid_check3/1(Signal)
  pCANR_kw_BMS2ChrgPwrAvail2/1 -> valid_check1/1(Signal)
  pHWIN_bool_BatSOHVld/1 -> valid_check7/2(Valid)
  pHWIN_bool_BatMaxTVld/1 -> valid_check8/2(Valid)
  pHWIN_bool_BatMinTVld/1 -> valid_check9/2(Valid)
  pHWIN_bool_BatAvgTVld/1 -> valid_check10/2(Valid)
  pHWIN_bool_BatInpTVld/1 -> valid_check11/2(Valid)
  pCANR_A_BMS1BatPackCurr/1 -> valid_check5/1(Signal)
  pCANR_pct_BMS3BatPackSOC/1 -> valid_check6/1(Signal)
  pCANR_pct_BMS3BatPackSOH/1 -> valid_check7/1(Signal)
  pCANR_degC_BMS5BatMaxTemp/1 -> valid_check8/1(Signal)
  pCANR_degC_BMS5BatMinTemp/1 -> valid_check9/1(Signal)
  pCANR_degC_BMS3BatPackTemp/1 -> valid_check10/1(Signal)
  pCANR_degC_BMS5BatInWaterTemp/1 -> valid_check11/1(Signal)
  valid_check5/1(SignalOut) -> pBMSI_A_BatActCurr/1
  valid_check6/1(SignalOut) -> pBMSI_pct_BatSOC/1, error_handling/2(BatStOfCh_p100)
  valid_check7/1(SignalOut) -> Terminator1/1
  valid_check8/1(SignalOut) -> pBMSI_degC_BatMaxTemp/1
  valid_check9/1(SignalOut) -> pBMSI_degC_BatMinTemp/1
  valid_check10/1(SignalOut) -> pBMSI_deg_BatAvgT/1
  valid_check11/1(SignalOut) -> pBMSI_degC_BatInpTemp/1
  pCANR_st_BMS1ChrgSt/1 -> pBMSI_st_BMSChrgSt/1, error_handling/1(BmsChrgSts_na)
  pCANR_bool_BMS1MainPlusCoilSt/1 -> pBMSI_bool_MainPosContaSt/1
  pCANR_bool_BMS1MainMinusCoilSt/1 -> pBMSI_bool_MainNegContaSt/1
  pCANR_bool_BMS1PreChrgCoilSt/1 -> pBMSI_bool_MainPreChrgContaSt/1
  pCANR_bool_BMS1ChrgReq/1 -> pBMSI_bool_BatChrgReq/1
  pHWIN_mV_IntlkA/1 -> interlock_check/1(InterlockA_mV)
  pHWIN_mV_IntlkB/1 -> interlock_check/2(InterlockB_mV)
  pCANR_st_BMS1BatPackSt/1 -> Convert7/1
  error_handling/1(BmsErr_na) -> pBMSI_st_BMSErr/1
  pCANR_st_BMS5IslaWarning/1 -> pBMSI_st_BatIslaMeasSt/1, error_handling/4(BatInsMeasSts_na)
  Convert7/1 -> error_handling/3(BmsSts_na), pBMSI_st_BMSSt/1
  error_handling1/1(DCChrgrErr_na) -> pBMSI_st_DCChrgrErr/1

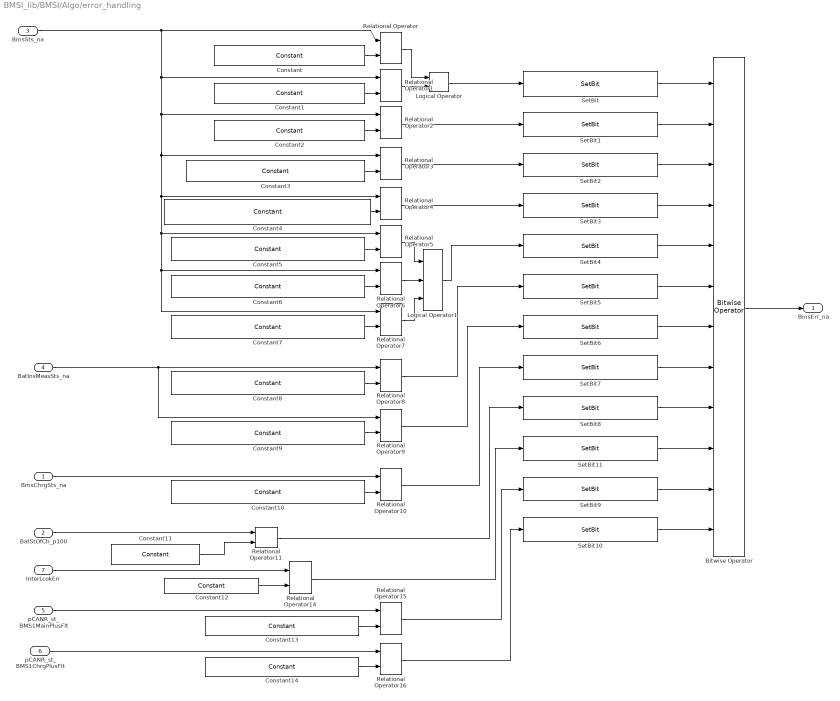
== system BMSI_lib/BMSI/Algo/error_handling ==
  BmsChrgSts_na : Inport  OutDataType=fixdt(1, 16)  OutScaling=2^0
  BatStOfCh_p100 : Inport  Port=2  OutDataType=fixdt(1, 16)  OutScaling=2^0
  BmsSts_na : Inport  Port=3  OutDataType=fixdt(1, 16)  OutScaling=2^0
  BatInsMeasSts_na : Inport  Port=4  OutDataType=fixdt(1, 16)  OutScaling=2^0
  pCANR_st_BMS1MainPlusFlt : Inport  Port=5  OutDataType=fixdt(1, 16)  OutScaling=2^0
  pCANR_st_BMS1ChrgPlusFlt : Inport  Port=6  OutDataType=fixdt(1, 16)  OutScaling=2^0
  InterLcokErr : Inport  Port=7  OutDataType=fixdt(1, 16)  OutScaling=2^0
  Bitwise Operator : BaseOperationLib_Browser/Others Unchanged/Bitwise Operator  logicop=OR  UseBitMask=off  NumInputPorts=12  BitMask=bin2dec('11011001')  BitMaskRealWorld=Stored Integer
  Constant : BaseOperationLib_Browser/Sources&Sinks/Constant  Value=uint8(FAWBMSStsTyp.WARN)  OutMin=[]  OutMax=[]  OutDataType=Enum: FAWBMSStsTyp  ConRadixGroup=Best Precision: Vector-wise  OutScaling=[]  OutDataTypeStr=Inherit: Inherit from 'Constant value'
  Constant1 : BaseOperationLib_Browser/Sources&Sinks/Constant  Value=uint8(FAWBMSStsTyp.WARN_DERATING)  OutMin=[]  OutMax=[]  OutDataType=Enum: FAWBMSStsTyp  ConRadixGroup=Best Precision: Vector-wise  OutScaling=[]  OutDataTypeStr=Inherit: Inherit from 'Constant value'
  Constant10 : BaseOperationLib_Browser/Sources&Sinks/Constant  Value=uint8(FAWBmsChrgStsTyp.CHARGING_FAULT)  OutMin=[]  OutMax=[]  OutDataType=Enum: FAWBmsChrgStsTyp  ConRadixGroup=Best Precision: Vector-wise  OutScaling=[]  OutDataTypeStr=Inherit: Inherit from 'Constant value'
  Constant11 : BaseOperationLib_Browser/Sources&Sinks/Constant  Value=pBMSI_pct_LoSOCThd_C  OutMin=[]  OutMax=[]  OutDataType=fixdt(1, 16)  ConRadixGroup=Use specified scaling  OutScaling=2^0  OutDataTypeStr=Inherit: Inherit from 'Constant value'
  Constant12 : BaseOperationLib_Browser/Sources&Sinks/Constant  Value=p_bool_True_M  OutMin=[]  OutMax=[]  OutDataType=fixdt(1, 16)  ConRadixGroup=Use specified scaling  OutScaling=2^0  OutDataTypeStr=Inherit: Inherit from 'Constant value'
  Constant13 : BaseOperationLib_Browser/Sources&Sinks/Constant  Value=uint8(FAWBmsContErrTyp.BMS_Cont_Normal)  OutMin=[]  OutMax=[]  OutDataTypeMode=uint8  OutDataType=fixdt(1, 16)  ConRadixGroup=Use specified scaling  OutScaling=2^0  OutDataTypeStr=uint8
  Constant14 : BaseOperationLib_Browser/Sources&Sinks/Constant  Value=uint8(FAWBmsContErrTyp.BMS_Cont_Normal)  OutMin=[]  OutMax=[]  OutDataTypeMode=uint8  OutDataType=fixdt(1, 16)  ConRadixGroup=Use specified scaling  OutScaling=2^0  OutDataTypeStr=uint8
  Constant2 : BaseOperationLib_Browser/Sources&Sinks/Constant  Value=uint8(FAWBMSStsTyp.FLT_UNABLE_CHARGING)  OutMin=[]  OutMax=[]  OutDataType=Enum: FAWBMSStsTyp  ConRadixGroup=Best Precision: Vector-wise  OutScaling=[]  OutDataTypeStr=Inherit: Inherit from 'Constant value'
  Constant3 : BaseOperationLib_Browser/Sources&Sinks/Constant  Value=uint8(FAWBMSStsTyp.FLT_UNABLE_DISCHARGING)  OutMin=[]  OutMax=[]  OutDataType=Enum: FAWBMSStsTyp  ConRadixGroup=Best Precision: Vector-wise  OutScaling=[]  OutDataTypeStr=Inherit: Inherit from 'Constant value'
  Constant4 : BaseOperationLib_Browser/Sources&Sinks/Constant  Value=uint8(FAWBMSStsTyp.CRITFLT_CHARGER_CONTACTORS_FAULT)  OutMin=[]  OutMax=[]  OutDataType=Enum: FAWBMSStsTyp  ConRadixGroup=Best Precision: Vector-wise  OutScaling=[]  OutDataTypeStr=Inherit: Inherit from 'Constant value'
  Constant5 : BaseOperationLib_Browser/Sources&Sinks/Constant  Value=uint8(FAWBMSStsTyp.CRITFLT_MAIN_CONTACTORS_FAULT)  OutMin=[]  OutMax=[]  OutDataType=Enum: FAWBMSStsTyp  ConRadixGroup=Best Precision: Vector-wise  OutScaling=[]  OutDataTypeStr=Inherit: Inherit from 'Constant value'
  Constant6 : BaseOperationLib_Browser/Sources&Sinks/Constant  Value=uint8(FAWBMSStsTyp.CRITFLT_CONTACTORS_OFF_BY_HCU)  OutMin=[]  OutMax=[]  OutDataType=Enum: FAWBMSStsTyp  ConRadixGroup=Best Precision: Vector-wise  OutScaling=[]  OutDataTypeStr=Inherit: Inherit from 'Constant value'
  Constant7 : BaseOperationLib_Browser/Sources&Sinks/Constant  Value=uint8(FAWBMSStsTyp.CRITFLT_CONTACTORS_OFF_BY_BMS)  OutMin=[]  OutMax=[]  OutDataType=Enum: FAWBMSStsTyp  ConRadixGroup=Best Precision: Vector-wise  OutScaling=[]  OutDataTypeStr=Inherit: Inherit from 'Constant value'
  Constant8 : BaseOperationLib_Browser/Sources&Sinks/Constant  Value=uint8(FAWBatInsMeasStsTyp.BIM_SECOND_LEVEL_WARNING)  OutMin=[]  OutMax=[]  OutDataType=Enum: FAWBatInsMeasStsTyp  ConRadixGroup=Best Precision: Vector-wise  OutScaling=[]  OutDataTypeStr=Inherit: Inherit from 'Constant value'
  Constant9 : BaseOperationLib_Browser/Sources&Sinks/Constant  Value=uint8(FAWBatInsMeasStsTyp.BIM_FIRST_LEVEL_WARNING)  OutMin=[]  OutMax=[]  OutDataType=Enum: FAWBatInsMeasStsTyp  ConRadixGroup=Best Precision: Vector-wise  OutScaling=[]  OutDataTypeStr=Inherit: Inherit from 'Constant value'
  Logical Operator : BaseOperationLib_Browser/Logic Operations Changed/Logical Operator  Operator=OR  Inputs=2  AllPortsSameDT=on  OutDataTypeMode=Specify via dialog  LogicDataType=PDT_Bool  OutDataTypeStr=PDT_Bool
  Logical Operator1 : BaseOperationLib_Browser/Logic Operations Changed/Logical Operator  Operator=OR  Inputs=3  AllPortsSameDT=on  OutDataTypeMode=Specify via dialog  LogicDataType=PDT_Bool  OutDataTypeStr=PDT_Bool
  Relational Operator{,1..10,14} (12 alike) : BaseOperationLib_Browser/Logic Operations Changed/Relational Operator  Operator===  InputSameDT=on  LogicOutDataTypeMode=Specify via dialog  LogicDataType=PDT_Bool  OutDataTypeStr=PDT_Bool
  Relational Operator11 : BaseOperationLib_Browser/Logic Operations Changed/Relational Operator  Operator=<=  InputSameDT=on  LogicOutDataTypeMode=Specify via dialog  LogicDataType=PDT_Bool  OutDataTypeStr=PDT_Bool
  Relational Operator15 : BaseOperationLib_Browser/Logic Operations Changed/Relational Operator  Operator=>  InputSameDT=on  LogicOutDataTypeMode=Specify via dialog  LogicDataType=PDT_Bool  OutDataTypeStr=PDT_Bool
  Relational Operator16 : BaseOperationLib_Browser/Logic Operations Changed/Relational Operator  Operator=>  InputSameDT=on  LogicOutDataTypeMode=Specify via dialog  LogicDataType=PDT_Bool  OutDataTypeStr=PDT_Bool
  SetBit : PES_CZ_FAW/Discontinuities/SetBit  SystemSampleTime=-1  maska=FAWBmsErrTyp.BMS_WARNING
  SetBit1 : PES_CZ_FAW/Discontinuities/SetBit  SystemSampleTime=-1  maska=FAWBmsErrTyp.BMS_CHARGING_ERROR
  SetBit10 : PES_CZ_FAW/Discontinuities/SetBit  SystemSampleTime=-1  maska=FAWBmsErrTyp.BMS_ChrgPlus_FAULT
  SetBit11 : PES_CZ_FAW/Discontinuities/SetBit  SystemSampleTime=-1  maska=FAWBmsErrTyp.InterLockErr
  SetBit2 : PES_CZ_FAW/Discontinuities/SetBit  SystemSampleTime=-1  maska=FAWBmsErrTyp.BMS_DISCHARGING_ERROR
  SetBit3 : PES_CZ_FAW/Discontinuities/SetBit  SystemSampleTime=-1  maska=FAWBmsErrTyp.BMS_DC_CHARGING_ERROR
  SetBit4 : PES_CZ_FAW/Discontinuities/SetBit  SystemSampleTime=-1  maska=FAWBmsErrTyp.BMS_CRITICAL_ERROR
  SetBit5 : PES_CZ_FAW/Discontinuities/SetBit  SystemSampleTime=-1  maska=FAWBmsErrTyp.IMCU_SECOND_LEVEL_WARNING
  SetBit6 : PES_CZ_FAW/Discontinuities/SetBit  SystemSampleTime=-1  maska=FAWBmsErrTyp.IMCU_FIRST_LEVEL_WARNING
  SetBit7 : PES_CZ_FAW/Discontinuities/SetBit  SystemSampleTime=-1  maska=FAWBmsErrTyp.BMS_CHARGING_FAULT
  SetBit8 : PES_CZ_FAW/Discontinuities/SetBit  SystemSampleTime=-1  maska=FAWBmsErrTyp.LOW_SOC
  SetBit9 : PES_CZ_FAW/Discontinuities/SetBit  SystemSampleTime=-1  maska=FAWBmsErrTyp.BMS_MainPlus_FAULT
  BmsErr_na : Outport  OutDataType=fixdt(1, 16)  OutScaling=2^0
  wires:
  Constant14/1 -> Relational Operator16/2
  Constant13/1 -> Relational Operator15/2
  Relational Operator16/1 -> SetBit10/1
  Relational Operator15/1 -> SetBit9/1
  Constant12/1 -> Relational Operator14/2
  InterLcokErr/1 -> Relational Operator14/1
  SetBit11/1 -> Bitwise Operator/10
  Relational Operator14/1 -> SetBit11/1
  pCANR_st_BMS1ChrgPlusFlt/1 -> Relational Operator16/1
  pCANR_st_BMS1MainPlusFlt/1 -> Relational Operator15/1
  SetBit10/1 -> Bitwise Operator/12
  SetBit9/1 -> Bitwise Operator/11
  SetBit/1 -> Bitwise Operator/1
  SetBit1/1 -> Bitwise Operator/2
  SetBit2/1 -> Bitwise Operator/3
  SetBit3/1 -> Bitwise Operator/4
  SetBit4/1 -> Bitwise Operator/5
  SetBit5/1 -> Bitwise Operator/6
  SetBit6/1 -> Bitwise Operator/7
  SetBit7/1 -> Bitwise Operator/8
  Bitwise Operator/1 -> BmsErr_na/1
  Constant/1 -> Relational Operator/2
  BmsSts_na/1 -> Relational Operator/1, Relational Operator1/1, Relational Operator2/1, Relational Operator3/1, Relational Operator4/1, Relational Operator5/1, Relational Operator7/1, Relational Operator6/1
  Constant1/1 -> Relational Operator1/2
  Relational Operator/1 -> Logical Operator/1
  Relational Operator1/1 -> Logical Operator/2
  Logical Operator/1 -> SetBit/1
  Constant2/1 -> Relational Operator2/2
  Relational Operator2/1 -> SetBit1/1
  Constant3/1 -> Relational Operator3/2
  Relational Operator3/1 -> SetBit2/1
  Constant4/1 -> Relational Operator4/2
  Relational Operator4/1 -> SetBit3/1
  Constant5/1 -> Relational Operator5/2
  Constant6/1 -> Relational Operator6/2
  Constant7/1 -> Relational Operator7/2
  Relational Operator5/1 -> Logical Operator1/1
  Relational Operator6/1 -> Logical Operator1/2
  Relational Operator7/1 -> Logical Operator1/3
  Logical Operator1/1 -> SetBit4/1
  BatInsMeasSts_na/1 -> Relational Operator8/1, Relational Operator9/1
  Constant8/1 -> Relational Operator8/2
  Relational Operator8/1 -> SetBit5/1
  Constant9/1 -> Relational Operator9/2
  Relational Operator9/1 -> SetBit6/1
  BmsChrgSts_na/1 -> Relational Operator10/1
  Constant10/1 -> Relational Operator10/2
  Relational Operator10/1 -> SetBit7/1
  BatStOfCh_p100/1 -> Relational Operator11/1
  Constant11/1 -> Relational Operator11/2
  SetBit8/1 -> Bitwise Operator/9
  Relational Operator11/1 -> SetBit8/1

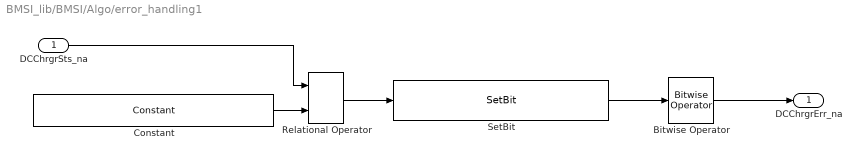
== system BMSI_lib/BMSI/Algo/error_handling1 ==
  DCChrgrSts_na : Inport  OutDataType=fixdt(1, 16)  OutScaling=2^0
  Bitwise Operator : BaseOperationLib_Browser/Others Unchanged/Bitwise Operator  logicop=OR  UseBitMask=off  BitMask=bin2dec('11011001')  BitMaskRealWorld=Stored Integer
  Constant : BaseOperationLib_Browser/Sources&Sinks/Constant  Value=pBMSI_st_DCChrgrErrSt_C  OutMin=[]  OutMax=[]  OutDataType=Enum: FAWBMSStsTyp  ConRadixGroup=Best Precision: Vector-wise  OutScaling=[]  OutDataTypeStr=Inherit: Inherit from 'Constant value'
  Relational Operator : BaseOperationLib_Browser/Logic Operations Changed/Relational Operator  Operator=>=  InputSameDT=on  LogicOutDataTypeMode=Specify via dialog  LogicDataType=PDT_Bool  OutDataTypeStr=PDT_Bool
  SetBit : PES_CZ_FAW/Discontinuities/SetBit  SystemSampleTime=-1  maska=FAWDCChrgrErr.FDC_DCChrgrErr
  DCChrgrErr_na : Outport  OutDataType=fixdt(1, 16)  OutScaling=2^0
  wires:
  SetBit/1 -> Bitwise Operator/1
  Bitwise Operator/1 -> DCChrgrErr_na/1
  Constant/1 -> Relational Operator/2
  DCChrgrSts_na/1 -> Relational Operator/1
  Relational Operator/1 -> SetBit/1

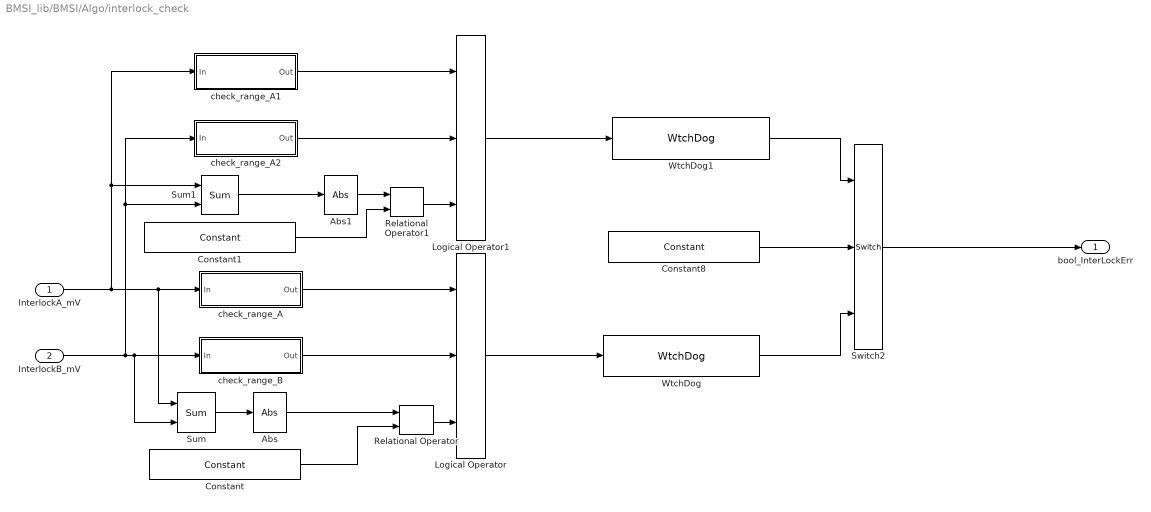
== system BMSI_lib/BMSI/Algo/interlock_check ==
  InterlockA_mV : Inport  OutDataType=fixdt(1, 16)  OutScaling=2^0
  InterlockB_mV : Inport  Port=2  OutDataType=fixdt(1, 16)  OutScaling=2^0
  Abs : BaseOperationLib_Browser/Math Operations Changed/Abs  OutMax=[]  OutDataType=fixdt(1, 16)  OutScaling=2^0  SaturateOnIntegerOverflow=on
  Abs1 : BaseOperationLib_Browser/Math Operations Changed/Abs  OutMax=[]  OutDataType=fixdt(1, 16)  OutScaling=2^0  SaturateOnIntegerOverflow=on
  Constant : BaseOperationLib_Browser/Sources&Sinks/Constant  Value=pBMSI_mV_InterlockDiffThd_C  OutMin=[]  OutMax=[]  OutDataType=fixdt(1, 16)  ConRadixGroup=Use specified scaling  OutScaling=2^0  OutDataTypeStr=Inherit: Inherit from 'Constant value'
  Constant1 : BaseOperationLib_Browser/Sources&Sinks/Constant  Value=pBMSI_mV_InterlockDiffThd_C  OutMin=[]  OutMax=[]  OutDataType=fixdt(1, 16)  ConRadixGroup=Use specified scaling  OutScaling=2^0  OutDataTypeStr=Inherit: Inherit from 'Constant value'
  Constant8 : BaseOperationLib_Browser/Sources&Sinks/Constant  Value=p_bool_dSPaceEnbl_C  OutMin=[]  OutMax=[]  OutDataType=fixdt(1, 16)  ConRadixGroup=Use specified scaling  OutScaling=2^0  OutDataTypeStr=Inherit: Inherit from 'Constant value'
  Logical Operator : BaseOperationLib_Browser/Logic Operations Changed/Logical Operator  Operator=AND  Inputs=3  AllPortsSameDT=on  OutDataTypeMode=Specify via dialog  LogicDataType=PDT_Bool  OutDataTypeStr=PDT_Bool
  Logical Operator1 : BaseOperationLib_Browser/Logic Operations Changed/Logical Operator  Operator=AND  Inputs=3  AllPortsSameDT=on  OutDataTypeMode=Specify via dialog  LogicDataType=PDT_Bool  OutDataTypeStr=PDT_Bool
  Relational Operator : BaseOperationLib_Browser/Logic Operations Changed/Relational Operator  Operator=<=  InputSameDT=on  LogicOutDataTypeMode=Specify via dialog  LogicDataType=PDT_Bool  OutDataTypeStr=PDT_Bool
  Relational Operator1 : BaseOperationLib_Browser/Logic Operations Changed/Relational Operator  Operator=<=  InputSameDT=on  LogicOutDataTypeMode=Specify via dialog  LogicDataType=PDT_Bool  OutDataTypeStr=PDT_Bool
  Sum : BaseOperationLib_Browser/Math Operations Changed/Sum  Inputs=+-  InputSameDT=on  OutMin=[]  OutMax=[]  OutDataType=fixdt(1, 16)  OutScaling=2^0  SaturateOnIntegerOverflow=on
  Sum1 : BaseOperationLib_Browser/Math Operations Changed/Sum  Inputs=+-  InputSameDT=on  OutMin=[]  OutMax=[]  OutDataType=fixdt(1, 16)  OutScaling=2^0  SaturateOnIntegerOverflow=on
  Switch2 : BaseOperationLib_Browser/Signal Routing Changed/Switch  Criteria=u2 ~= 0  Threshold=1  InputSameDT=on  OutMin=[]  OutMax=[]  OutDataType=fixdt(1,16,0)  OutScaling=[]  SaturateOnIntegerOverflow=on
  WtchDog : PES_CZ_FAW/Discontinuities/WtchDog  SystemSampleTime=-1  timeoutthres=pBMSI_s_TiDlyInterlockSts_C
  WtchDog1 : PES_CZ_FAW/Discontinuities/WtchDog  SystemSampleTime=-1  timeoutthres=pBMSI_s_TiDlyInterlockSts_C
  check_range_A : Subsystem
  check_range_A1 : Subsystem
  check_range_A2 : Subsystem
  check_range_B : Subsystem
  bool_InterLockErr : Outport  OutDataType=fixdt(1, 16)  OutScaling=2^0
  wires:
  Relational Operator/1 -> Logical Operator/3
  Constant/1 -> Relational Operator/2
  Abs/1 -> Relational Operator/1
  Sum/1 -> Abs/1
  check_range_A/1(Out) -> Logical Operator/1
  check_range_B/1(Out) -> Logical Operator/2
  InterlockB_mV/1 -> Sum/2, check_range_B/1(In), Sum1/2, check_range_A2/1(In)
  InterlockA_mV/1 -> Sum/1, check_range_A/1(In), check_range_A1/1(In), Sum1/1
  Logical Operator/1 -> WtchDog/1
  Constant8/1 -> Switch2/2
  Logical Operator1/1 -> WtchDog1/1
  WtchDog/1 -> Switch2/3
  Switch2/1 -> bool_InterLockErr/1
  check_range_A2/1(Out) -> Logical Operator1/2
  Sum1/1 -> Abs1/1
  check_range_A1/1(Out) -> Logical Operator1/1
  WtchDog1/1 -> Switch2/1
  Abs1/1 -> Relational Operator1/1
  Relational Operator1/1 -> Logical Operator1/3
  Constant1/1 -> Relational Operator1/2

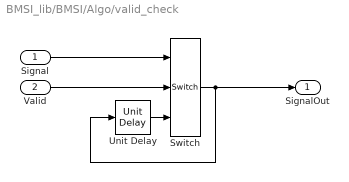
== system BMSI_lib/BMSI/Algo/valid_check ==
  Signal : Inport
  Valid : Inport  Port=2
  Switch : BaseOperationLib_Browser/Signal Routing Changed/Switch  Criteria=u2 ~= 0  Threshold=1  InputSameDT=on  OutMin=[]  OutMax=[]  OutDataType=fixdt(1,16,0)  OutScaling=[]  SaturateOnIntegerOverflow=on
  Unit Delay : BaseOperationLib_Browser/Discrete Unchanged /Unit Delay  X0=init  SampleTime=-1
  SignalOut : Outport
  wires:
  Switch/1 -> Unit Delay/1, SignalOut/1
  Unit Delay/1 -> Switch/3
  Signal/1 -> Switch/1
  Valid/1 -> Switch/2

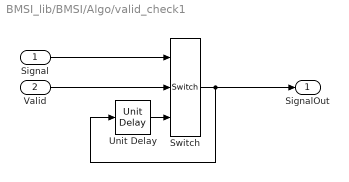
== system BMSI_lib/BMSI/Algo/valid_check1 ==
  Signal : Inport
  Valid : Inport  Port=2
  Switch : BaseOperationLib_Browser/Signal Routing Changed/Switch  Criteria=u2 ~= 0  Threshold=1  InputSameDT=on  OutMin=[]  OutMax=[]  OutDataType=fixdt(1,16,0)  OutScaling=[]  SaturateOnIntegerOverflow=on
  Unit Delay : BaseOperationLib_Browser/Discrete Unchanged /Unit Delay  X0=init  SampleTime=-1
  SignalOut : Outport
  wires:
  Valid/1 -> Switch/2
  Signal/1 -> Switch/1
  Unit Delay/1 -> Switch/3
  Switch/1 -> SignalOut/1, Unit Delay/1

== system BMSI_lib/BMSI/Algo/valid_check10 ==
  Signal : Inport
  Valid : Inport  Port=2
  Switch : BaseOperationLib_Browser/Signal Routing Changed/Switch  Criteria=u2 ~= 0  Threshold=1  InputSameDT=on  OutMin=[]  OutMax=[]  OutDataType=fixdt(1,16,0)  OutScaling=[]  SaturateOnIntegerOverflow=on
  Unit Delay : BaseOperationLib_Browser/Discrete Unchanged /Unit Delay  X0=init  SampleTime=-1
  SignalOut : Outport
  wires:
  Valid/1 -> Switch/2
  Signal/1 -> Switch/1
  Unit Delay/1 -> Switch/3
  Switch/1 -> SignalOut/1, Unit Delay/1

== system BMSI_lib/BMSI/Algo/valid_check11 ==
  Signal : Inport
  Valid : Inport  Port=2
  Switch : BaseOperationLib_Browser/Signal Routing Changed/Switch  Criteria=u2 ~= 0  Threshold=1  InputSameDT=on  OutMin=[]  OutMax=[]  OutDataType=fixdt(1,16,0)  OutScaling=[]  SaturateOnIntegerOverflow=on
  Unit Delay : BaseOperationLib_Browser/Discrete Unchanged /Unit Delay  X0=init  SampleTime=-1
  SignalOut : Outport
  wires:
  Valid/1 -> Switch/2
  Signal/1 -> Switch/1
  Unit Delay/1 -> Switch/3
  Switch/1 -> SignalOut/1, Unit Delay/1

== system BMSI_lib/BMSI/Algo/valid_check12 ==
  Signal : Inport
  Valid : Inport  Port=2
  Switch : BaseOperationLib_Browser/Signal Routing Changed/Switch  Criteria=u2 ~= 0  Threshold=1  InputSameDT=on  OutMin=[]  OutMax=[]  OutDataType=fixdt(1,16,0)  OutScaling=[]  SaturateOnIntegerOverflow=on
  Unit Delay : BaseOperationLib_Browser/Discrete Unchanged /Unit Delay  X0=init  SampleTime=-1
  SignalOut : Outport
  wires:
  Switch/1 -> Unit Delay/1, SignalOut/1
  Unit Delay/1 -> Switch/3
  Signal/1 -> Switch/1
  Valid/1 -> Switch/2

== system BMSI_lib/BMSI/Algo/valid_check13 ==
  Signal : Inport
  Valid : Inport  Port=2
  Switch : BaseOperationLib_Browser/Signal Routing Changed/Switch  Criteria=u2 ~= 0  Threshold=1  InputSameDT=on  OutMin=[]  OutMax=[]  OutDataType=fixdt(1,16,0)  OutScaling=[]  SaturateOnIntegerOverflow=on
  Unit Delay : BaseOperationLib_Browser/Discrete Unchanged /Unit Delay  X0=init  SampleTime=-1
  SignalOut : Outport
  wires:
  Valid/1 -> Switch/2
  Signal/1 -> Switch/1
  Unit Delay/1 -> Switch/3
  Switch/1 -> SignalOut/1, Unit Delay/1
